simulink model "ESC_cell_model"  (R2020b)
settings: Solver=VariableStepAuto  StartTime=0.0  StopTime=t_end  RelTol=1e-6
values from neighbouring files (symbols this model uses):
  A_an = 2.5e13    (= 25000000000000)    [main_cell.m]
  A_ca = 2.55e14    (= 255000000000000)    [main_cell.m]
  A_sei = 2.25e15    (= 2.25e+15)    [main_cell.m]
  A_surf = 0.009    [main_cell.m]
  alpha_cell = 1.1e-6    (= 1.1e-06)    [main_cell.m]
  capacity = 4.5    [Cell_1_RC_25.mat]    (also in Cell_43_RC_25.mat; parameters.mat = 10)
  DMC = [6.4338; 1413; -44.25]    [main_cell.m]
  E_an = 2.24e-19    [main_cell.m]
  E_ca = 2.64e-19    [main_cell.m]
  E_sei = 2.24e-19    [main_cell.m]
  EC = [6.4897; 1836.57; -102.23]    [main_cell.m]
  h_an = 1714*1000    (= 1714000)    [main_cell.m]
  h_ca = 790*1000    (= 790000)    [main_cell.m]
  h_sei = 257*1000    (= 257000)    [main_cell.m]
  k_b = 1.3806e-23    [main_cell.m]
  L = 2.4/1000    (= 0.0024)    [main_cell.m]
  m_an = 19.107/1000    (= 0.019107)    [main_cell.m]
  M_C6 = 72/1000    (= 0.072)    [main_cell.m]
  m_ca = 36.56/1000    (= 0.03656)    [main_cell.m]
  P_atm = 101e3    (= 101000)    [main_cell.m]
  P_crit = 158e3    (= 158000)    [main_cell.m]
  Q = capacity*3600*num_cells    [main.m]    (also in main_1S2P.m; main_cell.m = 4.6)
  R = 8.3145    [main_cell.m]
  R_ext = 0.002    [main.m]    (also in main_cell.m = 0.0066)
  R_tab = 0.0044    [main_cell.m]
  sigma_0 = data.Pressure(data_idx(1))-P_atm    [main_cell.m]
  SOC_0 = 1    [main.m]    (also in main_1S2P.m; main_cell.m)
  T_amb = data.CellTemperature(data_idx(1)) + 273.15    [main_cell.m]
  V_head_0 = 6.65e-6    (= 6.65e-06)    [main_cell.m]
  x_an_0 = 0.75    [main_cell.m]
  x_sei_0 = 0.15    [main_cell.m]
  y_dmc = 0.7    [main_cell.m]
  y_ec = 1-y_dmc    (= 0.3)    [main_cell.m]
  z_0 = 0.033    [main_cell.m]
libraries: fl_lib x21, nesl_utility x14, LiBatteryElements_lib x4, simulink x2
settings Model: Creator=Vivian  LastModifiedBy=Vivian
settings SolverCC: ZeroCrossAlgorithm=Adaptive
settings DebuggingCC: IgnoredZcDiagnostic=none

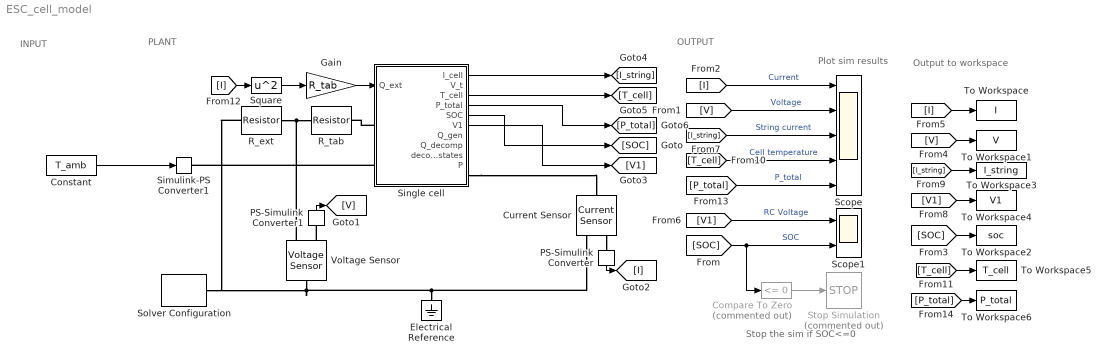
== system ESC_cell_model ==
  note: Output to workspace
  note: Plot sim results
  note: Stop the sim if SOC<=0
  note: PLANT
  note: INPUT
  note: OUTPUT
  Compare To Zero : simulink/Logic and Bit Operations/Compare To Zero  Commented=on  relop=<=  OutDataTypeStr=boolean
  Constant : Constant  Value=T_amb
  Current Sensor : fl_lib/Electrical/Electrical Sensors/Current Sensor
  Electrical Reference : fl_lib/Electrical/Electrical Elements/Electrical Reference
  Gain : Gain  Gain=R_tab
  PS-Simulink Converter : nesl_utility/PS-Simulink Converter  PhysicalDomain=network_engine_domain  SubClassName=ps_output  LeftPortType=input  RightPortType=output  PseudoPeriodic=off  Frequencies=[]  Unit=inherit  AffineConversion=off
  PS-Simulink Converter1 : nesl_utility/PS-Simulink Converter  PhysicalDomain=network_engine_domain  SubClassName=ps_output  LeftPortType=input  RightPortType=output  PseudoPeriodic=off  Frequencies=[]  Unit=inherit  AffineConversion=off
  R_ext : fl_lib/Electrical/Electrical Elements/Resistor  R=R_ext Ohm  i_specify=off  i_priority=None  i=0 A  i_nominal_specify=off  i_nominal_unit=A  i_nominal_value=1  v_specify=off  v_priority=None  v=0 V  v_nominal_specify=off  v_nominal_unit=V  v_nominal_value=1
  R_tab : fl_lib/Electrical/Electrical Elements/Resistor  R=R_tab Ohm  i_specify=off  i_priority=None  i=0 A  i_nominal_specify=off  i_nominal_unit=A  i_nominal_value=1  v_specify=off  v_priority=None  v=0 V  v_nominal_specify=off  v_nominal_unit=V  v_nominal_value=1
  Scope : Scope  NumInputPorts=5
  Scope1 : Scope  NumInputPorts=2
  Simulink-PS Converter1 : nesl_utility/Simulink-PS Converter  PhysicalDomain=network_engine_domain  SubClassName=ps_input  LeftPortType=input  RightPortType=output  PseudoPeriodic=off  Frequencies=[]  NoiseDistribution=none  NoiseParameters=[]  Unit=K  AffineConversion=off  FilteringAndDerivatives=provide  SimscapeFilterOrder=1  InputFilterTimeConstant=0.001  UdotUserProvided=0
  Single cell : Subsystem
  Solver Configuration : nesl_utility/Solver Configuration  PhysicalDomain=network_engine_domain  SubClassName=solver  LeftPortType=input  RightPortType=generic  Tones=[]  Harmonics=[]  SimulateNoise=off  Profile=off  UseLocalSampling=off  EnableSwitchedLinearOptims=on  FrequencyDomain=off  UseCCode=off  RelTol=0.001  AbsTol=1e-06  MinStep=1e-09  ToWorkspace=off  RevertToSquareIcSolve=off  NumHomotopyIterations=100  PhasorMode=off  PhasorModeNumHarmonics=1  DoDC=off  ResidualTolerance=1e-09  UseLocalSolver=off  LocalSolverChoice=NE_BACKWARD_EULER_ADVANCER  LocalSolverSampleTime=0.001  DoFixedCost=off  MaxNonlinIter=3  MaxModeIter=2  ComputeImpulses=off  ImpulseIterations=2  LinearAlgebra=auto  EquationFormulation=NE_TIME_EF  DelaysMemoryBudget=1024  AutomaticFiltering=on  FilteringTimeConstant=0.001  PartitionStorageMethod=AS_NEEDED  PartitionMemoryBudget=1024  PartitionMethod=ROBUST
  Square : Math  Operator=square  SaturateOnIntegerOverflow=on
  Stop Simulation : Stop  Commented=on
  To Workspace : ToWorkspace  VariableName=I  SaveFormat=Timeseries  SampleTime=-1
  To Workspace1 : ToWorkspace  VariableName=V  SaveFormat=Timeseries  SampleTime=-1
  To Workspace2 : ToWorkspace  VariableName=soc  SaveFormat=Timeseries  SampleTime=-1
  To Workspace3 : ToWorkspace  VariableName=I_string  SaveFormat=Timeseries  SampleTime=-1
  To Workspace4 : ToWorkspace  VariableName=V1  SaveFormat=Timeseries  SampleTime=-1
  To Workspace5 : ToWorkspace  VariableName=T_cell  SaveFormat=Timeseries  SampleTime=-1
  To Workspace6 : ToWorkspace  VariableName=P_total  SaveFormat=Timeseries  SampleTime=-1
  Voltage Sensor : fl_lib/Electrical/Electrical Sensors/Voltage Sensor
  wires:
  Compare To Zero/1 -> Stop Simulation/1
  Single cell/5(SOC) -> [SOC]
  [SOC] -> Compare To Zero/1, Scope1/2  "SOC"
  [V] -> Scope/2  "Voltage"
  PS-Simulink Converter/1 -> [I]
  PS-Simulink Converter1/1 -> [V]
  [I] -> Scope/1  "Current"
  [I] -> To Workspace/1
  [V] -> To Workspace1/1
  [SOC] -> To Workspace2/1
  Constant/1 -> Simulink-PS Converter1/1
  Single cell/6(V1) -> [V1]
  Single cell/1(I_cell) -> [I_string]
  [V1] -> To Workspace4/1
  [I_string] -> To Workspace3/1
  [V1] -> Scope1/1  "RC Voltage"
  Single cell/3(T_cell) -> [T_cell]
  [I_string] -> Scope/3  "String current"
  [T_cell] -> To Workspace5/1
  [I] -> Square/1
  Square/1 -> Gain/1
  Gain/1 -> Single cell/1(Q_ext)
  [T_cell] -> Scope/4  "Cell temperature"
  Single cell/4(P_total) -> [P_total]
  [P_total] -> Scope/5  "P_total"
  [P_total] -> To Workspace6/1
  connections:
  Current Sensor/RConn2 -- Electrical Reference/LConn1 -- R_ext/LConn1 -- Solver Configuration/RConn1 -- Voltage Sensor/LConn1
  Voltage Sensor/RConn1 -- PS-Simulink Converter1/LConn1
  Single cell/LConn1 -- R_tab/RConn1
  Single cell/RConn1 -- Current Sensor/LConn1
  Current Sensor/RConn1 -- PS-Simulink Converter/LConn1
  Single cell/LConn2 -- Simulink-PS Converter1/RConn1
  R_ext/RConn1 -- Voltage Sensor/RConn2 -- R_tab/LConn1

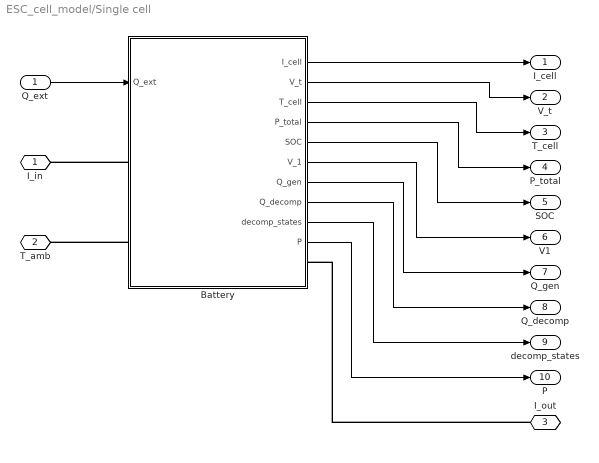
== system ESC_cell_model/Single cell ==
  Q_ext : Inport
  Battery : Subsystem
  I_in : PMIOPort  Side=Left
  T_amb : PMIOPort  Port=2  Side=Left
  I_out : PMIOPort  Port=3  Side=Right
  I_cell : Outport
  V_t : Outport  Port=2
  T_cell : Outport  Port=3
  P_total : Outport  Port=4
  SOC : Outport  Port=5
  V1 : Outport  Port=6
  Q_gen : Outport  Port=7
  Q_decomp : Outport  Port=8
  decomp_states : Outport  Port=9
  P : Outport  Port=10
  wires:
  Q_ext/1 -> Battery/1(Q_ext)
  Battery/1(I_cell) -> I_cell/1
  Battery/2(V_t) -> V_t/1
  Battery/3(T_cell) -> T_cell/1
  Battery/4(P_total) -> P_total/1
  Battery/5(SOC) -> SOC/1
  Battery/6(V_1) -> V1/1
  Battery/7(Q_gen) -> Q_gen/1
  Battery/8(Q_decomp) -> Q_decomp/1
  Battery/10(P) -> P/1
  Battery/9(decomp_states) -> decomp_states/1
  connections:
  Battery/LConn1 -- I_in/RConn1
  Battery/LConn2 -- T_amb/RConn1
  I_out/RConn1 -- Battery/RConn1

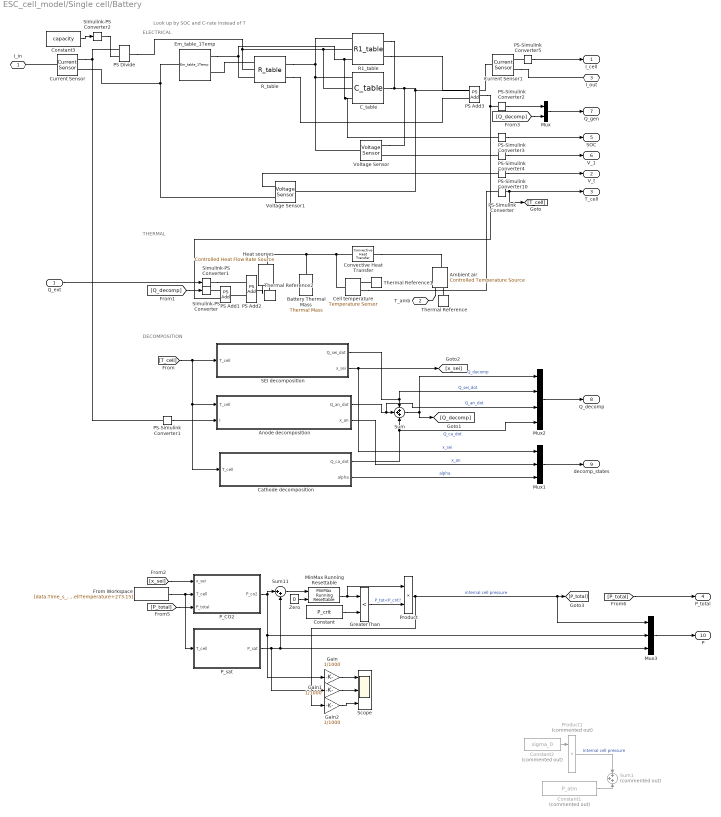
== system ESC_cell_model/Single cell/Battery ==
  note: Look up by SOC and C-rate instead of T
  note: DECOMPOSITION
  note: THERMAL
  note: ELECTRICAL
  Q_ext : Inport
  Ambient air : fl_lib/Thermal/Thermal Sources/Controlled Temperature Source
  Anode decomposition : Subsystem
  Battery Thermal Mass : fl_lib/Thermal/Thermal Elements/Thermal Mass  mass=cell_mass kg  sp_heat=cell_Cp_heat J/kg/K  T_specify=on  T_priority=High  T=T_amb K  T_nominal_specify=off  T_nominal_unit=K  T_nominal_value=1  Q_specify=on  Q_priority=None  Q=0 W  Q_nominal_specify=off  Q_nominal_unit=W  Q_nominal_value=1
  C_table : LiBatteryElements_lib/C_table  C_Table=C1 F  SOC_Table=SOC_RC  Temp_Table=T_RC degC  v0=0 V
      settings: SourceProductBaseCode=SS  InternalSimscapePortConfiguration="{\"Bottom\":[],\"Left\":[{\"id\":\"p\",\"label\":\"+\",\"type\":\"foundation.electrical.electrical\"},{\"id\":\"T\",\"label\":\"T\",\"type\":\"input\"},{\"id\":\"SOC\",\"label\":\"SOC\",\"type\":\"input\"}],\"Right\":[{\"id\":\"n\",\"label\":\"-\",\"type\":\"foundation.electrical.electrical\"}],\"Top\":[]}"
  Cathode decomposition : Subsystem
  Cell temperature : fl_lib/Thermal/Thermal Sensors/Temperature Sensor
  Constant : Constant  Value=P_crit
  Constant1 : Constant  Commented=on  Value=P_atm
  Constant2 : Constant  Commented=on  Value=sigma_0
  Constant3 : Constant  Value=capacity
  Convective Heat Transfer : fl_lib/Thermal/Thermal Elements/Convective Heat Transfer  area=cell_area m^2  heat_tr_coeff=h_conv W/(m^2 * K)  T_specify=off  T_priority=None  T=0 K  T_nominal_specify=off  T_nominal_unit=K  T_nominal_value=1  Q_specify=off  Q_priority=None  Q=0 W  Q_nominal_specify=off  Q_nominal_unit=W  Q_nominal_value=1
  Current Sensor : fl_lib/Electrical/Electrical Sensors/Current Sensor
  Current Sensor1 : fl_lib/Electrical/Electrical Sensors/Current Sensor
  Em_table_1Temp : LiBatteryElements_lib/Em_table_1Temp  Em_Table=OCV V  SOC_Table=SOC_OCV  C=Q hr*A  Qinit=(1-SOC_0)*Q hr*A
      settings: SourceProductBaseCode=SS  InternalSimscapePortConfiguration="{\"Bottom\":[],\"Left\":[{\"id\":\"p\",\"label\":\"+\",\"type\":\"foundation.electrical.electrical\"},{\"id\":\"SOC\",\"label\":\"SOC\",\"type\":\"output\"}],\"Right\":[{\"id\":\"n\",\"label\":\"-\",\"type\":\"foundation.electrical.electrical\"}],\"Top\":[]}"
  From Workspace : FromWorkspace  VariableName=[data.Time_s_, data.CellTemperature+273.15]
  Gain : Gain  Gain=1/1000
  Gain1 : Gain  Gain=1/1000
  Gain2 : Gain  Gain=1/1000
  GreaterThan : RelationalOperator  Operator=<  OutDataTypeStr=boolean  RndMeth=Simplest
  Heat sources : fl_lib/Thermal/Thermal Sources/Controlled Heat Flow Rate Source
  MinMax Running Resettable : simulink/Math Operations/MinMax Running Resettable  Function=max  vinit=0
  Mux : Mux  Inputs=2
  Mux1 : Mux  Inputs=3
  Mux2 : Mux
  Mux3 : Mux  Inputs=3
  PS Add1 : fl_lib/Physical Signals/Functions/PS Add
  PS Add2 : fl_lib/Physical Signals/Functions/PS Add
  PS Add3 : fl_lib/Physical Signals/Functions/PS Add
  PS Divide : fl_lib/Physical Signals/Functions/PS Divide
      settings: SourceProductBaseCode=SS
  PS-Simulink Converter{,1..5,10} (7 alike) : nesl_utility/PS-Simulink Converter  PhysicalDomain=network_engine_domain  SubClassName=ps_output  LeftPortType=input  RightPortType=output  PseudoPeriodic=off  Frequencies=[]  Unit=inherit  AffineConversion=off
  P_CO2 : Subsystem
  P_sat : Subsystem
  Product : Product
  Product1 : Product  Commented=on
  R1_table : LiBatteryElements_lib/R1_table  R_Table=R1 Ohm  SOC_Table=SOC_RC  Temp_Table=T_RC degC
      settings: SourceProductBaseCode=SS  InternalSimscapePortConfiguration="{\"Bottom\":[],\"Left\":[{\"id\":\"p\",\"label\":\"+\",\"type\":\"foundation.electrical.electrical\"},{\"id\":\"T\",\"label\":\"T\",\"type\":\"input\"},{\"id\":\"SOC\",\"label\":\"SOC\",\"type\":\"input\"}],\"Right\":[{\"id\":\"n\",\"label\":\"-\",\"type\":\"foundation.electrical.electrical\"},{\"id\":\"pow\",\"label\":\"POW\",\"type\":\"output\"}],\"Top\":[]}"
  R_table : LiBatteryElements_lib/R_table  R_Table=Rs Ohm  SOC_Table=SOC_RC  Temp_Table=T_RC degC
      settings: SourceProductBaseCode=SS  InternalSimscapePortConfiguration="{\"Bottom\":[],\"Left\":[{\"id\":\"p\",\"label\":\"+\",\"type\":\"foundation.electrical.electrical\"},{\"id\":\"T\",\"label\":\"T\",\"type\":\"input\"},{\"id\":\"SOC\",\"label\":\"SOC\",\"type\":\"input\"}],\"Right\":[{\"id\":\"n\",\"label\":\"-\",\"type\":\"foundation.electrical.electrical\"},{\"id\":\"pow\",\"label\":\"POW\",\"type\":\"output\"}],\"Top\":[]}"
  SEI decomposition : Subsystem
  Scope : Scope  NumInputPorts=3
  Simulink-PS Converter : nesl_utility/Simulink-PS Converter  PhysicalDomain=network_engine_domain  SubClassName=ps_input  LeftPortType=input  RightPortType=output  PseudoPeriodic=off  Frequencies=[]  NoiseDistribution=none  NoiseParameters=[]  Unit=W  AffineConversion=off  FilteringAndDerivatives=provide  SimscapeFilterOrder=1  InputFilterTimeConstant=0.001  UdotUserProvided=0
  Simulink-PS Converter1 : nesl_utility/Simulink-PS Converter  PhysicalDomain=network_engine_domain  SubClassName=ps_input  LeftPortType=input  RightPortType=output  PseudoPeriodic=off  Frequencies=[]  NoiseDistribution=none  NoiseParameters=[]  Unit=W  AffineConversion=off  FilteringAndDerivatives=provide  SimscapeFilterOrder=1  InputFilterTimeConstant=0.001  UdotUserProvided=0
  Simulink-PS Converter2 : nesl_utility/Simulink-PS Converter  PhysicalDomain=network_engine_domain  SubClassName=ps_input  LeftPortType=input  RightPortType=output  PseudoPeriodic=off  Frequencies=[]  NoiseDistribution=none  NoiseParameters=[]  Unit=A  AffineConversion=off  FilteringAndDerivatives=provide  SimscapeFilterOrder=1  InputFilterTimeConstant=0.001  UdotUserProvided=0
  Sum : Sum  Inputs=+++
  Sum1 : Sum  Commented=on  Inputs=+++
  Sum11 : Sum  Inputs=|++
  Thermal Reference : fl_lib/Thermal/Thermal Elements/Thermal Reference
  Thermal Reference1 : fl_lib/Thermal/Thermal Elements/Thermal Reference
  Thermal Reference2 : fl_lib/Thermal/Thermal Elements/Thermal Reference
  Voltage Sensor : fl_lib/Electrical/Electrical Sensors/Voltage Sensor
  Voltage Sensor1 : fl_lib/Electrical/Electrical Sensors/Voltage Sensor
  Zero : Constant  Value=0  OutDataTypeStr=Inherit: Inherit via back propagation
  I_in : PMIOPort  Side=Left
  T_amb : PMIOPort  Port=2  Side=Left
  I_out : PMIOPort  Port=3  Side=Right
  I_cell : Outport
  V_t : Outport  Port=2
  T_cell : Outport  Port=3
  P_total : Outport  Port=4
  SOC : Outport  Port=5
  V_1 : Outport  Port=6
  Q_gen : Outport  Port=7
  Q_decomp : Outport  Port=8
  decomp_states : Outport  Port=9
  P : Outport  Port=10
  wires:
  PS-Simulink Converter/1 -> T_cell/1, [T_cell]
  [Q_decomp] -> Simulink-PS Converter/1
  [T_cell] -> Cathode decomposition/1(T_cell), Anode decomposition/1(T_cell), SEI decomposition/1(T_cell)
  Anode decomposition/1(Q_an_dot) -> Sum/2, Mux2/3  "Q_an_dot"
  SEI decomposition/1(Q_sei_dot) -> Mux2/2, Sum/1  "Q_sei_dot"
  Cathode decomposition/1(Q_ca_dot) -> Sum/3, Mux2/4  "Q_ca_dot"
  SEI decomposition/2(x_sei) -> Mux1/1, [x_sei]  "x_sei"
  Anode decomposition/2(x_an) -> Mux1/2  "x_an"
  Cathode decomposition/2(alpha) -> Mux1/3  "alpha"
  Q_ext/1 -> Simulink-PS Converter1/1
  PS-Simulink Converter1/1 -> Anode decomposition/2(I)
  Sum11/1 -> MinMax Running Resettable/1
  [x_sei] -> P_CO2/1(x_sei)
  [P_total] -> P_CO2/3(P_total)
  P_CO2/1(P_co2) -> Gain/1, Mux3/2, Sum11/1
  From Workspace/1 -> P_sat/1(T_cell), P_CO2/2(T_cell)
  P_sat/1(P_sat) -> Gain1/1, Sum11/2, Mux3/3
  Constant/1 -> GreaterThan/2
  GreaterThan/1 -> Product/2  "P_tot<P_crit?"
  MinMax Running Resettable/1 -> Product/1, GreaterThan/1
  Zero/1 -> MinMax Running Resettable/2
  PS-Simulink Converter10/1 -> V_t/1
  PS-Simulink Converter4/1 -> V_1/1
  PS-Simulink Converter3/1 -> SOC/1
  PS-Simulink Converter5/1 -> I_cell/1
  Sum/1 -> Mux2/1, [Q_decomp]  "Q_decomp"
  PS-Simulink Converter2/1 -> Mux/1
  [Q_decomp] -> Mux/2
  Mux/1 -> Q_gen/1
  Mux1/1 -> decomp_states/1
  Mux2/1 -> Q_decomp/1
  Mux3/1 -> P/1
  [P_total] -> P_total/1
  Product/1 -> Gain2/1, Mux3/1, [P_total]  "internal cell pressure"
  Gain/1 -> Scope/1
  Gain1/1 -> Scope/2
  ? -> Product1/2  "P_tot<P_crit?"
  Constant1/1 -> Sum1/3
  Constant2/1 -> Product1/1
  Product1/1 -> Sum1/1  "Internal cell pressure"
  Gain2/1 -> Scope/3
  Constant3/1 -> Simulink-PS Converter2/1
  connections:
  PS-Simulink Converter4/LConn1 -- Voltage Sensor/RConn1
  PS-Simulink Converter10/LConn1 -- Voltage Sensor1/RConn1
  Voltage Sensor1/RConn2 -- Em_table_1Temp/RConn1 -- Current Sensor/RConn2
  R1_table/RConn1 -- C_table/RConn1 -- Voltage Sensor/RConn2 -- Current Sensor1/LConn1 -- Voltage Sensor1/LConn1
  Cell temperature/LConn1 -- Convective Heat Transfer/LConn1 -- Heat sources/LConn1 -- Battery Thermal Mass/LConn1
  Convective Heat Transfer/RConn1 -- Ambient air/LConn1
  Ambient air/RConn1 -- T_amb/RConn1
  Thermal Reference/LConn1 -- Ambient air/RConn2
  Thermal Reference1/LConn1 -- Cell temperature/RConn1
  Thermal Reference2/LConn1 -- Heat sources/RConn2
  PS Add1/LConn1 -- Simulink-PS Converter/RConn1
  PS Add2/LConn2 -- PS Add1/RConn1
  Heat sources/RConn1 -- PS Add2/RConn1
  Simulink-PS Converter1/RConn1 -- PS Add2/LConn1
  Current Sensor/LConn1 -- I_in/RConn1
  Current Sensor/RConn1 -- PS Divide/LConn1 -- PS-Simulink Converter1/LConn1
  Current Sensor1/RConn2 -- I_out/RConn1
  PS-Simulink Converter5/LConn1 -- Current Sensor1/RConn1
  R_table/RConn2 -- PS Add3/LConn2
  PS Add3/RConn1 -- PS Add1/LConn2 -- PS-Simulink Converter2/LConn1
  R1_table/RConn2 -- PS Add3/LConn1
  C_table/LConn1 -- Voltage Sensor/LConn1 -- R1_table/LConn1 -- R_table/RConn1
  R_table/LConn1 -- Em_table_1Temp/LConn1
  R_table/LConn3 -- Em_table_1Temp/LConn2 -- PS-Simulink Converter3/LConn1 -- C_table/LConn3 -- R1_table/LConn3
  Simulink-PS Converter2/RConn1 -- PS Divide/LConn2
  PS Divide/RConn1 -- R_table/LConn2 -- R1_table/LConn2 -- C_table/LConn2
  Cell temperature/RConn2 -- PS-Simulink Converter/LConn1

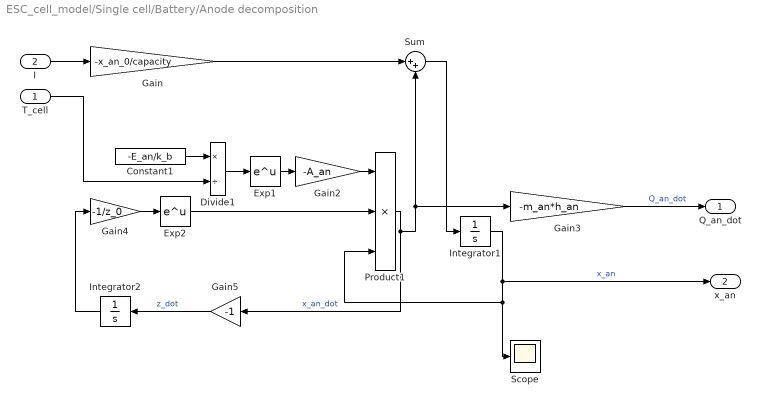
== system ESC_cell_model/Single cell/Battery/Anode decomposition ==
  T_cell : Inport
  I : Inport  Port=2
  Constant1 : Constant  Value=-E_an/k_b
  Divide1 : Product  Inputs=*/
  Exp1 : Math  SaturateOnIntegerOverflow=on
  Exp2 : Math  SaturateOnIntegerOverflow=on
  Gain : Gain  Gain=-x_an_0/capacity
  Gain2 : Gain  Gain=-A_an
  Gain3 : Gain  Gain=-m_an*h_an
  Gain4 : Gain  Gain=-1/z_0
  Gain5 : Gain  Gain=-1
  Integrator1 : Integrator  InitialCondition=x_an_0  LimitOutput=on  UpperSaturationLimit=x_an_0  LowerSaturationLimit=0
  Integrator2 : Integrator  InitialCondition=z_0  LimitOutput=on  LowerSaturationLimit=0
  Product1 : Product  Inputs=3
  Scope : Scope
  Sum : Sum  Inputs=|++
  Q_an_dot : Outport
  x_an : Outport  Port=2
  wires:
  Gain2/1 -> Product1/1
  Product1/1 -> Gain5/1, Sum/2, Gain3/1  "x_an_dot"
  Gain5/1 -> Integrator2/1  "z_dot"
  Divide1/1 -> Exp1/1
  Integrator2/1 -> Gain4/1
  Exp1/1 -> Gain2/1
  Integrator1/1 -> Scope/1, Product1/3, x_an/1  "x_an"
  Gain4/1 -> Exp2/1
  Constant1/1 -> Divide1/1
  Exp2/1 -> Product1/2
  Gain3/1 -> Q_an_dot/1  "Q_an_dot"
  T_cell/1 -> Divide1/2
  I/1 -> Gain/1
  Gain/1 -> Sum/1
  Sum/1 -> Integrator1/1

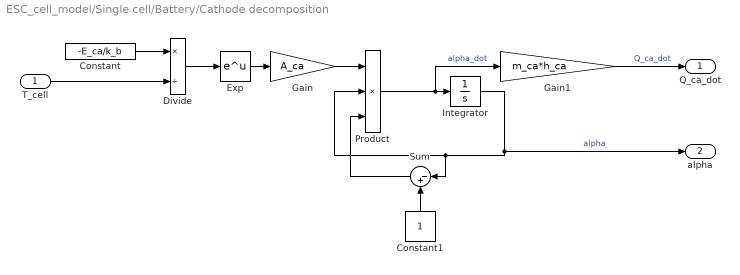
== system ESC_cell_model/Single cell/Battery/Cathode decomposition ==
  T_cell : Inport
  Constant : Constant  Value=-E_ca/k_b
  Constant1 : Constant
  Divide : Product  Inputs=*/
  Exp : Math  SaturateOnIntegerOverflow=on
  Gain : Gain  Gain=A_ca
  Gain1 : Gain  Gain=m_ca*h_ca
  Integrator : Integrator  InitialCondition=x_sei_0  LimitOutput=on  UpperSaturationLimit=x_sei_0  LowerSaturationLimit=0
  Product : Product  Inputs=3
  Sum : Sum  Inputs=|-+
  Q_ca_dot : Outport
  alpha : Outport  Port=2
  wires:
  Constant/1 -> Divide/1
  Product/1 -> Gain1/1, Integrator/1  "alpha_dot"
  Gain1/1 -> Q_ca_dot/1  "Q_ca_dot"
  Integrator/1 -> Sum/1, Product/2, alpha/1  "alpha"
  Gain/1 -> Product/1
  T_cell/1 -> Divide/2
  Divide/1 -> Exp/1
  Exp/1 -> Gain/1
  Constant1/1 -> Sum/2
  Sum/1 -> Product/3

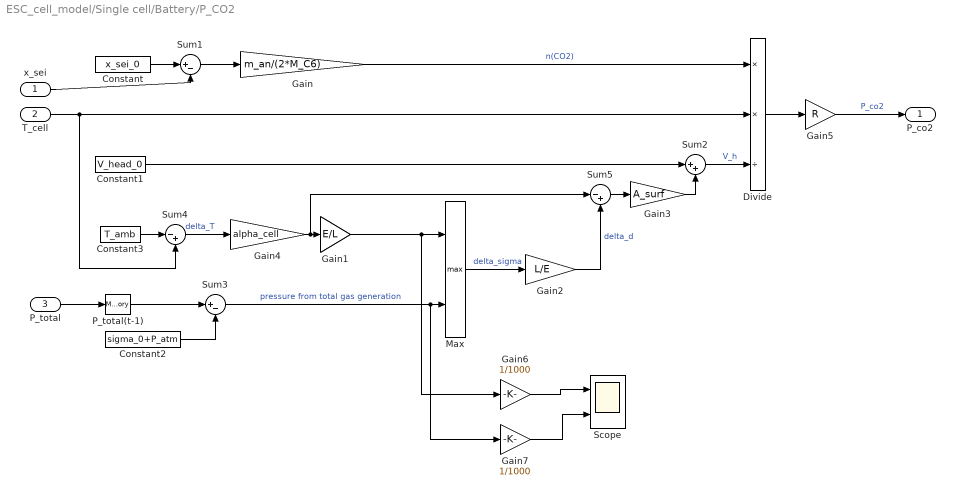
== system ESC_cell_model/Single cell/Battery/P_CO2 ==
  x_sei : Inport
  T_cell : Inport  Port=2
  P_total : Inport  Port=3
  Constant : Constant  Value=x_sei_0
  Constant1 : Constant  Value=V_head_0
  Constant2 : Constant  Value=sigma_0+P_atm
  Constant3 : Constant  Value=T_amb
  Divide : Product  Inputs=**/
  Gain : Gain  Gain=m_an/(2*M_C6)
  Gain1 : Gain  Gain=E/L
  Gain2 : Gain  Gain=L/E
  Gain3 : Gain  Gain=A_surf
  Gain4 : Gain  Gain=alpha_cell
  Gain5 : Gain  Gain=R
  Gain6 : Gain  Gain=1/1000
  Gain7 : Gain  Gain=1/1000
  Max : MinMax  Function=max  Inputs=2
  P_total(t-1) : Memory  InitialCondition=sigma_0 + P_atm
  Scope : Scope  NumInputPorts=2
  Sum1 : Sum  Inputs=|+-
  Sum2 : Sum  Inputs=|++
  Sum3 : Sum  Inputs=|+-
  Sum4 : Sum  Inputs=|-+
  Sum5 : Sum  Inputs=|-+
  P_co2 : Outport
  wires:
  Sum4/1 -> Gain4/1  "delta_T"
  Gain2/1 -> Sum5/2  "delta_d"
  Constant1/1 -> Sum2/1
  Sum1/1 -> Gain/1
  T_cell/1 -> Divide/2, Sum4/2
  Divide/1 -> Gain5/1
  Sum5/1 -> Gain3/1
  Max/1 -> Gain2/1  "delta_sigma"
  Gain4/1 -> Sum5/1, Gain1/1
  P_total/1 -> P_total(t-1)/1
  P_total(t-1)/1 -> Sum3/1
  Gain5/1 -> P_co2/1  "P_co2"
  Constant2/1 -> Sum3/2
  Constant/1 -> Sum1/1
  Sum3/1 -> Gain7/1, Max/2  "pressure from total gas generation"
  Gain3/1 -> Sum2/2
  Gain/1 -> Divide/1  "n(CO2)"
  Sum2/1 -> Divide/3  "V_h"
  Constant3/1 -> Sum4/1
  x_sei/1 -> Sum1/2
  Gain6/1 -> Scope/1
  Gain7/1 -> Scope/2
  Gain1/1 -> Gain6/1, Max/1

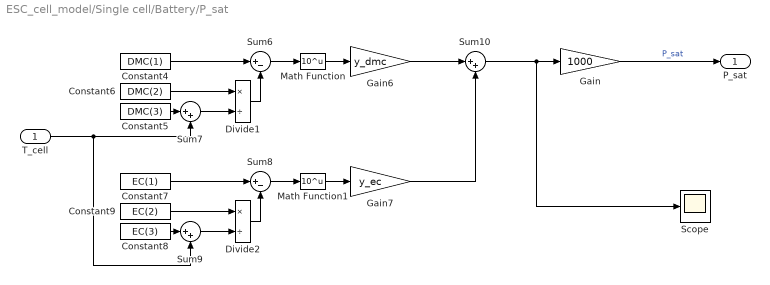
== system ESC_cell_model/Single cell/Battery/P_sat ==
  T_cell : Inport
  Constant4 : Constant  Value=DMC(1)
  Constant5 : Constant  Value=DMC(3)
  Constant6 : Constant  Value=DMC(2)
  Constant7 : Constant  Value=EC(1)
  Constant8 : Constant  Value=EC(3)
  Constant9 : Constant  Value=EC(2)
  Divide1 : Product  Inputs=*/
  Divide2 : Product  Inputs=*/
  Gain : Gain  Gain=1000
  Gain6 : Gain  Gain=y_dmc
  Gain7 : Gain  Gain=y_ec
  Math Function : Math  Operator=10^u  SaturateOnIntegerOverflow=on
  Math Function1 : Math  Operator=10^u  SaturateOnIntegerOverflow=on
  Scope : Scope
  Sum10 : Sum  Inputs=|++
  Sum6 : Sum  Inputs=|+-
  Sum7 : Sum  Inputs=|++
  Sum8 : Sum  Inputs=|+-
  Sum9 : Sum  Inputs=|++
  P_sat : Outport
  wires:
  Constant7/1 -> Sum8/1
  Math Function1/1 -> Gain7/1
  Sum9/1 -> Divide2/2
  Sum6/1 -> Math Function/1
  Sum7/1 -> Divide1/2
  Divide2/1 -> Sum8/2
  T_cell/1 -> Sum9/2, Sum7/2
  Constant4/1 -> Sum6/1
  Math Function/1 -> Gain6/1
  Constant8/1 -> Sum9/1
  Sum8/1 -> Math Function1/1
  Constant9/1 -> Divide2/1
  Divide1/1 -> Sum6/2
  Constant5/1 -> Sum7/1
  Constant6/1 -> Divide1/1
  Gain6/1 -> Sum10/1
  Gain7/1 -> Sum10/2
  Sum10/1 -> Scope/1, Gain/1
  Gain/1 -> P_sat/1  "P_sat"

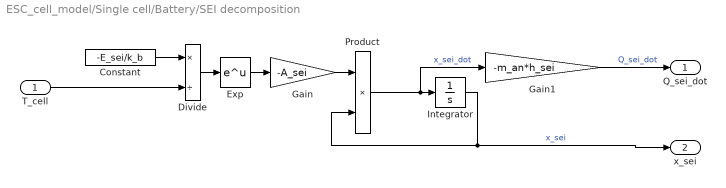
== system ESC_cell_model/Single cell/Battery/SEI decomposition ==
  T_cell : Inport
  Constant : Constant  Value=-E_sei/k_b
  Divide : Product  Inputs=*/
  Exp : Math  SaturateOnIntegerOverflow=on
  Gain : Gain  Gain=-A_sei
  Gain1 : Gain  Gain=-m_an*h_sei
  Integrator : Integrator  InitialCondition=x_sei_0  LimitOutput=on  UpperSaturationLimit=x_sei_0  LowerSaturationLimit=0
  Product : Product
  Q_sei_dot : Outport
  x_sei : Outport  Port=2
  wires:
  Constant/1 -> Divide/1
  Product/1 -> Gain1/1, Integrator/1  "x_sei_dot"
  Gain1/1 -> Q_sei_dot/1  "Q_sei_dot"
  Integrator/1 -> x_sei/1, Product/2  "x_sei"
  Gain/1 -> Product/1
  T_cell/1 -> Divide/2
  Divide/1 -> Exp/1
  Exp/1 -> Gain/1
